simulink library "INT_PTODi_TrqLeadCoord"  (R2016b)
settings: Solver=VariableStepAuto  StartTime=0.0  StopTime=10.0  RelTol=1e-3
settings Model: Creator=Administrator  LastModifiedBy=Administrator

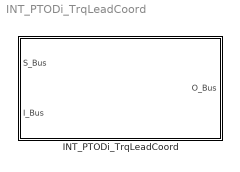
== system INT_PTODi_TrqLeadCoord ==
  INT_PTODi_TrqLeadCoord : Subsystem

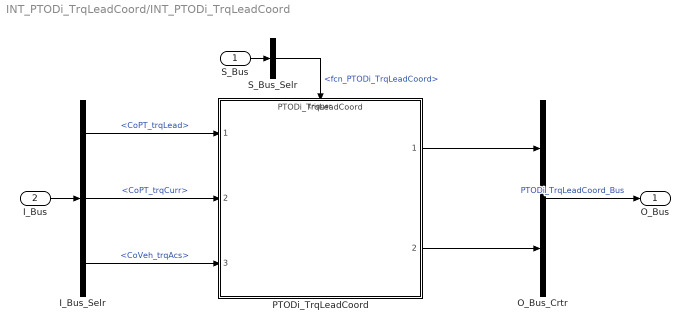
== system INT_PTODi_TrqLeadCoord/INT_PTODi_TrqLeadCoord ==
  S_Bus : Inport
  I_Bus : Inport  Port=2
  I_Bus_Selr : BusSelector  OutputSignals=CoPT_trqLead,CoPT_trqCurr,CoVeh_trqAcs
  O_Bus_Crtr : BusCreator  Inputs=2
  PTODi_TrqLeadCoord : ModelReference  ModelNameDialog=PTODi_TrqLeadCoord  SimulationMode=Normal  ModelReferenceVersion=1.3  TriggerPortName=function  TriggerPortTriggerType=function-call  TriggerPortStatesWhenEnabling=held
  S_Bus_Selr : BusSelector  OutputSignals=fcn_PTODi_TrqLeadCoord
  O_Bus : Outport
  wires:
  S_Bus_Selr/1 -> PTODi_TrqLeadCoord/Trigger  "<fcn_PTODi_TrqLeadCoord>"
  S_Bus/1 -> S_Bus_Selr/1
  I_Bus/1 -> I_Bus_Selr/1
  I_Bus_Selr/1 -> PTODi_TrqLeadCoord/1  "<CoPT_trqLead>"
  I_Bus_Selr/2 -> PTODi_TrqLeadCoord/2  "<CoPT_trqCurr>"
  I_Bus_Selr/3 -> PTODi_TrqLeadCoord/3  "<CoVeh_trqAcs>"
  O_Bus_Crtr/1 -> O_Bus/1  "PTODi_TrqLeadCoord_Bus"
  PTODi_TrqLeadCoord/1 -> O_Bus_Crtr/1
  PTODi_TrqLeadCoord/2 -> O_Bus_Crtr/2
